simulink model "MarchMPC"  (R2024a)
settings: Solver=daessc  StartTime=0.0  StopTime=15  FixedStep=0.01  RelTol=1e-3
undefined symbols (not defined in the file): dw_des, leg_controller, LFstates, LRstates, model, p_cur, p_des, param, px, py, pz, Q, RFstates, RRstates, v_cur, v_des, vx, vy, vz, w, w_des, X, Y, Z
libraries: sm_lib x57, nesl_utility x47
(part 1 of 4)
settings Model: Creator=a123  LastModifiedBy=a123
settings RTWCC: GPUComputeCapability=3.5

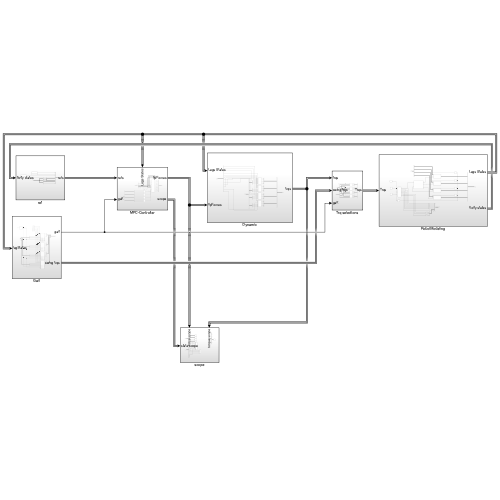
[thumbnail: Simulink's stored preview of the top-level diagram]
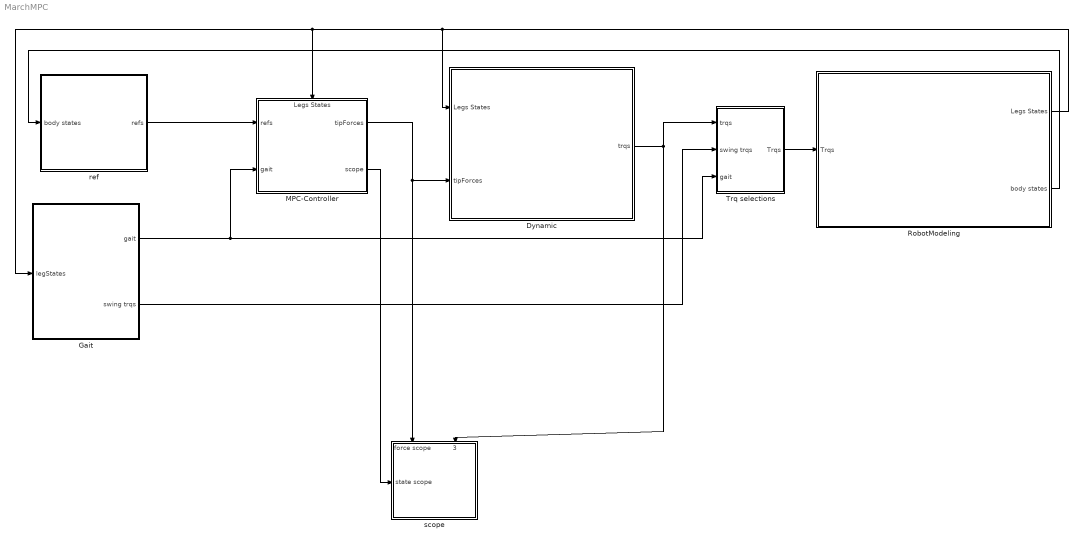
== system MarchMPC ==
  Dynamic : Subsystem
  Gait : Subsystem
  MPC-Controller : Subsystem
      settings: PortSchema="{\"entries\":[{\"content\":{\"sides\":[{\"content\":{\"connectorIds\":[\"In1\",\"In2\"]},\"type\":\"ConnectorPlacement.EquallySpacedRectSide\",\"uuid\":\"82207ac2-498d-428d-bb4d-b0457fff2070\"},{\"content\":{\"connectorIds\":[\"Out1\",\"Out2\"],\"side\":\"RIGHT\"},\"type\":\"ConnectorPlacement.EquallySpacedRectSide\",\"uuid\":\"62017463-8491-4b37-95c8-f619666068a7\"},{\"content\":{\"connectorIds\":[\"In3\"],\"side\":\"TOP\"},\"type\":\"ConnectorPlacement.EquallySpacedRectSide\",\"uuid\":\"cf9993cf-df0f-41a3-a963-d91c0f700b7a\"}]},\"type\":\"ConnectorPlacement.EquallySpacedConnector\",\"uuid\":\"3cbcd1c8-4438-4464-bb77-c195fb75fbb3\"}],\"packageUris\":[\"http://schema.mathworks.com/mf0/Connector/R2020b\"],\"version\":\"1.0\"}"
  RobotModeling : Subsystem
  Trq selections : Subsystem
  ref : Subsystem
  scope : Subsystem
      settings: PortSchema="{\"entries\":[{\"content\":{\"sides\":[{\"content\":{\"connectorIds\":[\"In1\"]},\"type\":\"ConnectorPlacement.EquallySpacedRectSide\",\"uuid\":\"c0265f70-bade-488b-ae2d-3c8d38e3d5ac\"},{\"content\":{\"side\":\"RIGHT\"},\"type\":\"ConnectorPlacement.EquallySpacedRectSide\",\"uuid\":\"4660b7bc-d16b-42a4-852b-cf8f48253a71\"},{\"content\":{\"connectorIds\":[\"In2\",\"In3\"],\"side\":\"TOP\"},\"type\":\"ConnectorPlacement.EquallySpacedRectSide\",\"uuid\":\"c4e122d6-8b41-4744-828b-3ddf3ee2b8ae\"}]},\"type\":\"ConnectorPlacement.EquallySpacedConnector\",\"uuid\":\"80d21178-9509-4fd6-959c-ba40dd2e55fa\"}],\"packageUris\":[\"http://schema.mathworks.com/mf0/Connector/R2020b\"],\"version\":\"1.0\"}"
  wires:
  RobotModeling/2(" body states") -> ref/1(body states)
  Dynamic/1(trqs) -> Trq selections/1(trqs), scope/3(torque scope)
  RobotModeling/1(Legs States) -> Dynamic/1(Legs States), MPC-Controller/3(Legs States), Gait/1(legStates)
  ref/1(refs) -> MPC-Controller/1(refs)
  Gait/1(gait) -> Trq selections/3(gait), MPC-Controller/2(gait)
  MPC-Controller/2(scope) -> scope/1(state scope)
  MPC-Controller/1(tipForces) -> Dynamic/2(tipForces), scope/2(force scope)
  Gait/2(swing trqs) -> Trq selections/2(swing trqs)
  Trq selections/1(Trqs) -> RobotModeling/1(Trqs)

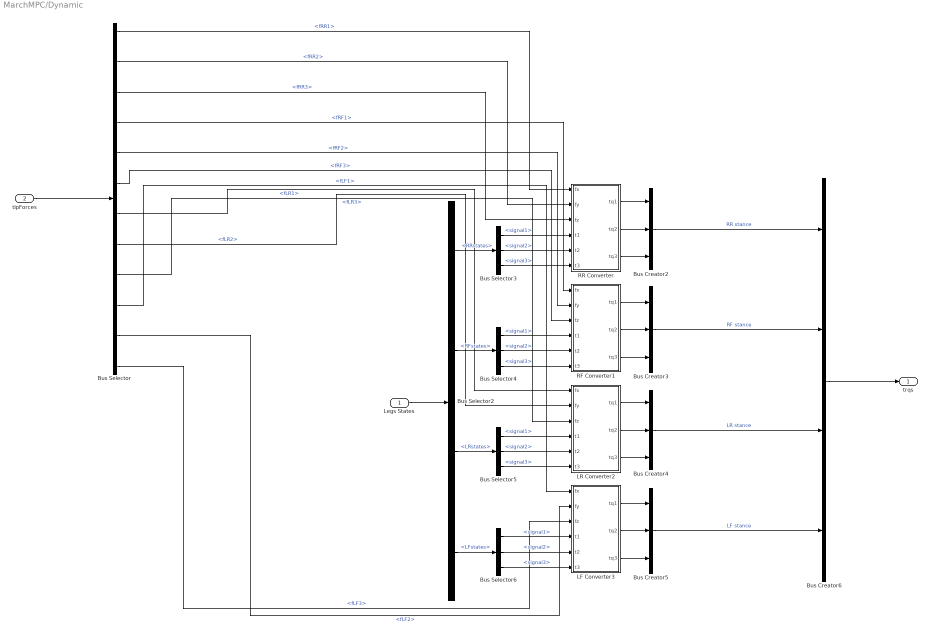
== system MarchMPC/Dynamic ==
  Legs States : Inport
  tipForces : Inport  Port=2
  Bus Creator{2..5} (4 alike) : BusCreator  Inputs=3
  Bus Creator6 : BusCreator  Inputs=4
  Bus Selector : BusSelector  OutputSignals=fRR1,fRR2,fRR3,fRF1,fRF2,fRF3,fLR1,fLR2,fLR3,fLF1,fLF2,fLF3
  Bus Selector2 : BusSelector  OutputSignals=RRstates,RFstates,LRstates,LFstates
  Bus Selector{3..6} (4 alike) : BusSelector  OutputSignals=signal1,signal2,signal3
  LF Converter3 : MATLAB Function  TreatAsAtomicUnit=on
  LR Converter2 : MATLAB Function  TreatAsAtomicUnit=on
  RF Converter1 : MATLAB Function  TreatAsAtomicUnit=on
  RR Converter : MATLAB Function  TreatAsAtomicUnit=on
  trqs : Outport
  wires:
  Bus Creator2/1 -> Bus Creator6/1  "RR stance"
  Bus Creator3/1 -> Bus Creator6/2  "RF stance"
  Bus Creator4/1 -> Bus Creator6/3  "LR stance"
  Bus Creator5/1 -> Bus Creator6/4  "LF stance"
  Bus Creator6/1 -> trqs/1
  Legs States/1 -> Bus Selector2/1
  Bus Selector2/1 -> Bus Selector3/1  "<RRstates>"
  Bus Selector3/1 -> RR Converter/4(t1)  "<signal1>"
  Bus Selector3/2 -> RR Converter/5(t2)  "<signal2>"
  Bus Selector3/3 -> RR Converter/6(t3)  "<signal3>"
  Bus Selector2/2 -> Bus Selector4/1  "<RFstates>"
  Bus Selector2/3 -> Bus Selector5/1  "<LRstates>"
  Bus Selector2/4 -> Bus Selector6/1  "<LFstates>"
  Bus Selector4/1 -> RF Converter1/4(t1)  "<signal1>"
  Bus Selector4/2 -> RF Converter1/5(t2)  "<signal2>"
  Bus Selector4/3 -> RF Converter1/6(t3)  "<signal3>"
  Bus Selector5/1 -> LR Converter2/4(t1)  "<signal1>"
  Bus Selector5/2 -> LR Converter2/5(t2)  "<signal2>"
  Bus Selector5/3 -> LR Converter2/6(t3)  "<signal3>"
  Bus Selector6/1 -> LF Converter3/4(t1)  "<signal1>"
  Bus Selector6/2 -> LF Converter3/5(t2)  "<signal2>"
  Bus Selector6/3 -> LF Converter3/6(t3)  "<signal3>"
  RR Converter/3(tq3) -> Bus Creator2/3
  RR Converter/2(tq2) -> Bus Creator2/2
  RR Converter/1(tq1) -> Bus Creator2/1
  RF Converter1/1(tq1) -> Bus Creator3/1
  RF Converter1/2(tq2) -> Bus Creator3/2
  RF Converter1/3(tq3) -> Bus Creator3/3
  LR Converter2/1(tq1) -> Bus Creator4/1
  LR Converter2/2(tq2) -> Bus Creator4/2
  LR Converter2/3(tq3) -> Bus Creator4/3
  LF Converter3/1(tq1) -> Bus Creator5/1
  LF Converter3/2(tq2) -> Bus Creator5/2
  LF Converter3/3(tq3) -> Bus Creator5/3
  tipForces/1 -> Bus Selector/1
  Bus Selector/1 -> RR Converter/1(fx)  "<fRR1>"
  Bus Selector/2 -> RR Converter/2(fy)  "<fRR2>"
  Bus Selector/3 -> RR Converter/3(fz)  "<fRR3>"
  Bus Selector/4 -> RF Converter1/1(fx)  "<fRF1>"
  Bus Selector/5 -> RF Converter1/2(fy)  "<fRF2>"
  Bus Selector/6 -> RF Converter1/3(fz)  "<fRF3>"
  Bus Selector/7 -> LR Converter2/1(fx)  "<fLR1>"
  Bus Selector/8 -> LR Converter2/2(fy)  "<fLR2>"
  Bus Selector/9 -> LR Converter2/3(fz)  "<fLR3>"
  Bus Selector/10 -> LF Converter3/1(fx)  "<fLF1>"
  Bus Selector/11 -> LF Converter3/2(fy)  "<fLF2>"
  Bus Selector/12 -> LF Converter3/3(fz)  "<fLF3>"

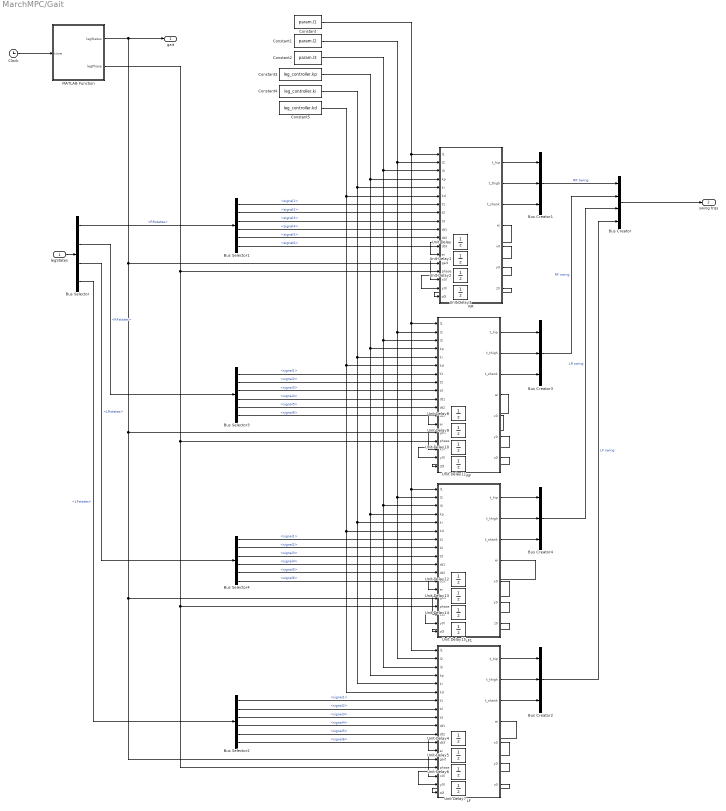
== system MarchMPC/Gait ==
  legStates : Inport
  Bus Creator : BusCreator  Inputs=RR Swing,RF swing,LR swing,LF swing
  Bus Creator{1..4} (4 alike) : BusCreator  Inputs=3
  Bus Selector : BusSelector  OutputSignals=RRstates,RFstates,LRstates,LFstates
  Bus Selector{1..4} (4 alike) : BusSelector  OutputSignals=signal1,signal2,signal3,signal4,signal5,signal6
  Clock : Clock
  Constant : Constant  Value=param.l1
  Constant1 : Constant  Value=param.l2
  Constant2 : Constant  Value=param.l3
  Constant3 : Constant  Value=leg_controller.kp
  Constant4 : Constant  Value=leg_controller.ki
  Constant5 : Constant  Value=leg_controller.kd
  LF : MATLAB Function  TreatAsAtomicUnit=on
  LF1 : MATLAB Function  TreatAsAtomicUnit=on
  MATLAB Function : MATLAB Function  TreatAsAtomicUnit=on
  RF : MATLAB Function  TreatAsAtomicUnit=on
  RR : MATLAB Function  TreatAsAtomicUnit=on
  Unit Delay{,4,8,12} (4 alike) : UnitDelay  InitialCondition=[0 0 0]  SampleTime=-1  HasFrameUpgradeWarning=on
  Unit Delay{1..3,5..7,9..11,13..15} (12 alike) : UnitDelay  SampleTime=-1  HasFrameUpgradeWarning=on
  gait : Outport
  swing trqs : Outport  Port=2
  wires:
  Clock/1 -> MATLAB Function/1(time)
  legStates/1 -> Bus Selector/1
  Bus Selector/1 -> Bus Selector1/1  "<RRstates>"
  RR/2(t_thigh) -> Bus Creator1/2
  RR/3(t_shank) -> Bus Creator1/3
  Bus Selector1/3 -> RR/9(t3)  "<signal3>"
  Bus Creator1/1 -> Bus Creator/1  "RR Swing"
  Bus Selector1/1 -> RR/7(t1)  "<signal1>"
  Bus Selector1/6 -> RR/12(dt3)  "<signal6>"
  Bus Selector1/5 -> RR/11(dt2)  "<signal5>"
  RR/1(t_hip) -> Bus Creator1/1
  Bus Selector1/2 -> RR/8(t2)  "<signal2>"
  Unit Delay/1 -> RR/13("ei ")
  Bus Selector1/4 -> RR/10(dt1)  "<signal4>"
  RR/4(ei) -> Unit Delay/1
  Bus Creator/1 -> swing trqs/1
  RR/5(x0) -> Unit Delay1/1
  Unit Delay1/1 -> RR/16(x0l)
  RR/6(y0) -> Unit Delay2/1
  Unit Delay2/1 -> RR/17(y0l)
  RR/7(z0) -> Unit Delay3/1
  Unit Delay3/1 -> RR/18(z0l)
  Unit Delay4/1 -> LF/13("ei ")
  LF/2(t_thigh) -> Bus Creator2/2
  LF/1(t_hip) -> Bus Creator2/1
  Unit Delay6/1 -> LF/17(y0l)
  LF/3(t_shank) -> Bus Creator2/3
  LF/4(ei) -> Unit Delay4/1
  Bus Creator2/1 -> Bus Creator/4  "LF swing"
  Bus Selector2/1 -> LF/7(t1)  "<signal1>"
  Bus Selector2/5 -> LF/11(dt2)  "<signal5>"
  Bus Selector2/2 -> LF/8(t2)  "<signal2>"
  Bus Selector2/3 -> LF/9(t3)  "<signal3>"
  LF/5(x0) -> Unit Delay5/1
  Bus Selector2/4 -> LF/10(dt1)  "<signal4>"
  Bus Selector2/6 -> LF/12(dt3)  "<signal6>"
  LF/6(y0) -> Unit Delay6/1
  Unit Delay7/1 -> LF/18(z0l)
  LF/7(z0) -> Unit Delay7/1
  Unit Delay5/1 -> LF/16(x0l)
  Bus Selector/4 -> Bus Selector2/1  "<LFstates>"
  Unit Delay8/1 -> RF/13("ei ")
  Bus Selector/2 -> Bus Selector3/1  "<RFstates>"
  Bus Selector3/1 -> RF/7(t1)  "<signal1>"
  RF/2(t_thigh) -> Bus Creator3/2
  RF/1(t_hip) -> Bus Creator3/1
  Unit Delay10/1 -> RF/17(y0l)
  MATLAB Function/1(legStatus) -> gait/1, LF/14(gait), LF1/14(gait), RF/14(gait), RR/14(gait)
  Bus Selector3/5 -> RF/11(dt2)  "<signal5>"
  MATLAB Function/2(legPhase) -> LF/15(phase), LF1/15(phase), RF/15(phase), RR/15(phase)
  Bus Selector3/2 -> RF/8(t2)  "<signal2>"
  Bus Selector3/3 -> RF/9(t3)  "<signal3>"
  RF/5(x0) -> Unit Delay9/1
  Bus Selector3/4 -> RF/10(dt1)  "<signal4>"
  RF/4(ei) -> Unit Delay8/1
  RF/3(t_shank) -> Bus Creator3/3
  Bus Selector3/6 -> RF/12(dt3)  "<signal6>"
  RF/6(y0) -> Unit Delay10/1
  Unit Delay11/1 -> RF/18(z0l)
  RF/7(z0) -> Unit Delay11/1
  Unit Delay9/1 -> RF/16(x0l)
  Bus Creator3/1 -> Bus Creator/2  "RF swing"
  Bus Selector/3 -> Bus Selector4/1  "<LRstates>"
  LF1/1(t_hip) -> Bus Creator4/1
  Unit Delay13/1 -> LF1/16(x0l)
  Unit Delay14/1 -> LF1/17(y0l)
  LF1/2(t_thigh) -> Bus Creator4/2
  Bus Selector4/1 -> LF1/7(t1)  "<signal1>"
  Bus Selector4/2 -> LF1/8(t2)  "<signal2>"
  Bus Selector4/3 -> LF1/9(t3)  "<signal3>"
  Unit Delay15/1 -> LF1/18(z0l)
  Bus Selector4/4 -> LF1/10(dt1)  "<signal4>"
  LF1/5(x0) -> Unit Delay13/1
  LF1/3(t_shank) -> Bus Creator4/3
  LF1/4(ei) -> Unit Delay12/1
  LF1/7(z0) -> Unit Delay15/1
  LF1/6(y0) -> Unit Delay14/1
  Bus Selector4/6 -> LF1/12(dt3)  "<signal6>"
  Bus Selector4/5 -> LF1/11(dt2)  "<signal5>"
  Unit Delay12/1 -> LF1/13("ei ")
  Bus Creator4/1 -> Bus Creator/3  "LR swing"
  Constant/1 -> RR/1(l1), LF/1(l1), LF1/1(l1), RF/1(l1)
  Constant1/1 -> RR/2(l2), LF/2(l2), LF1/2(l2), RF/2(l2)
  Constant2/1 -> RR/3(l3), LF/3(l3), LF1/3(l3), RF/3(l3)
  Constant3/1 -> LF/4(kp), LF1/4(kp), RF/4(kp), RR/4(kp)
  Constant4/1 -> LF/5(ki), LF1/5(ki), RF/5(ki), RR/5(ki)
  Constant5/1 -> LF/6(kd), LF1/6(kd), RF/6(kd), RR/6(kd)

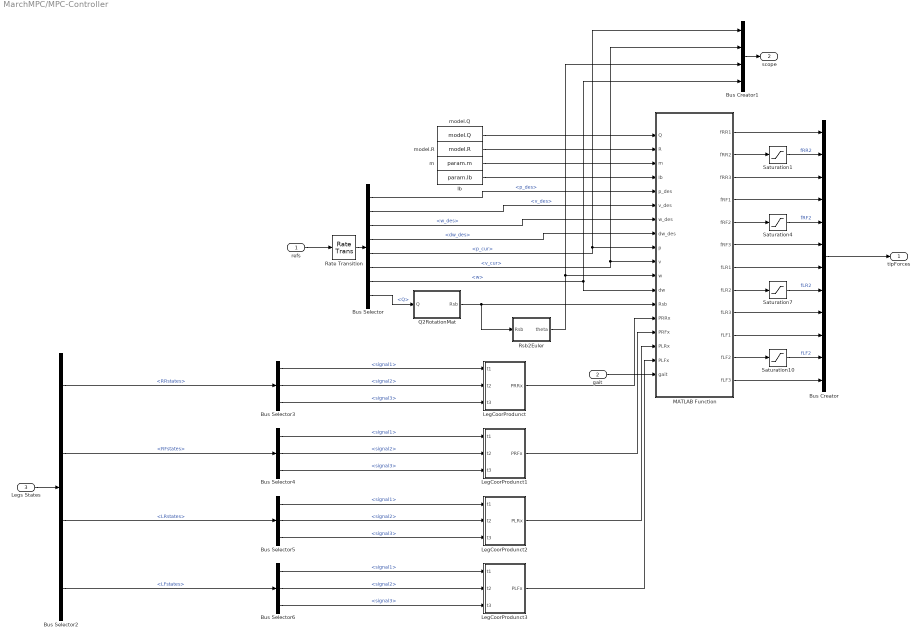
== system MarchMPC/MPC-Controller ==
  refs : Inport
  gait : Inport  Port=2
  Legs States : Inport  Port=3
  Bus Creator : BusCreator  Inputs=12
  Bus Creator1 : BusCreator  Inputs=4
  Bus Selector : BusSelector  OutputSignals=p_des,v_des,w_des,dw_des,p_cur,v_cur,w,Q
  Bus Selector2 : BusSelector  OutputSignals=RRstates,RFstates,LRstates,LFstates
  Bus Selector{3..6} (4 alike) : BusSelector  OutputSignals=signal1,signal2,signal3
  Ib : Constant  Value=param.Ib  VectorParams1D=off
  LegCoorProdunct : MATLAB Function  TreatAsAtomicUnit=on
  LegCoorProdunct1 : MATLAB Function  TreatAsAtomicUnit=on
  LegCoorProdunct2 : MATLAB Function  TreatAsAtomicUnit=on
  LegCoorProdunct3 : MATLAB Function  TreatAsAtomicUnit=on
  MATLAB Function : MATLAB Function  TreatAsAtomicUnit=on
  Q2RotationMat : MATLAB Function  TreatAsAtomicUnit=on
  Rate Transition : RateTransition  OutPortSampleTime=0.01
  Rsb2Euler : MATLAB Function  TreatAsAtomicUnit=on
  Saturation{1,4,7,10} (4 alike) : Saturate  UpperLimit=200  LowerLimit=0
  m : Constant  Value=param.m
  model.Q : Constant  Value=model.Q  VectorParams1D=off
  model.R : Constant  Value=model.R  VectorParams1D=off
  tipForces : Outport
  scope : Outport  Port=2
  wires:
  refs/1 -> Rate Transition/1
  Bus Selector/1 -> MATLAB Function/5(p_des)  "<p_des>"
  Bus Selector/2 -> MATLAB Function/6(v_des)  "<v_des>"
  Bus Selector/3 -> MATLAB Function/7(w_des)  "<w_des>"
  Bus Selector/4 -> MATLAB Function/8(dw_des)  "<dw_des>"
  Bus Selector/5 -> Bus Creator1/1, MATLAB Function/9(p)  "<p_cur>"
  Bus Selector/6 -> Bus Creator1/2, MATLAB Function/10(v)  "<v_cur>"
  Bus Selector/7 -> Bus Creator1/4, MATLAB Function/12(dw)  "<w>"
  Bus Selector/8 -> Q2RotationMat/1(Q)  "<Q>"
  Bus Selector5/2 -> LegCoorProdunct2/2(t2)  "<signal2>"
  Bus Selector5/3 -> LegCoorProdunct2/3(t3)  "<signal3>"
  Bus Selector6/3 -> LegCoorProdunct3/3(t3)  "<signal3>"
  Bus Selector2/3 -> Bus Selector5/1  "<LRstates>"
  Bus Selector6/1 -> LegCoorProdunct3/1(t1)  "<signal1>"
  Bus Selector4/2 -> LegCoorProdunct1/2(t2)  "<signal2>"
  Bus Selector6/2 -> LegCoorProdunct3/2(t2)  "<signal2>"
  Bus Selector3/2 -> LegCoorProdunct/2(t2)  "<signal2>"
  Bus Selector5/1 -> LegCoorProdunct2/1(t1)  "<signal1>"
  Bus Selector2/2 -> Bus Selector4/1  "<RFstates>"
  Bus Selector2/1 -> Bus Selector3/1  "<RRstates>"
  Legs States/1 -> Bus Selector2/1
  Bus Selector3/3 -> LegCoorProdunct/3(t3)  "<signal3>"
  Bus Selector4/1 -> LegCoorProdunct1/1(t1)  "<signal1>"
  Bus Selector3/1 -> LegCoorProdunct/1(t1)  "<signal1>"
  Bus Selector4/3 -> LegCoorProdunct1/3(t3)  "<signal3>"
  Bus Selector2/4 -> Bus Selector6/1  "<LFstates>"
  Bus Creator/1 -> tipForces/1
  Q2RotationMat/1(Rsb) -> Rsb2Euler/1(Rsb), MATLAB Function/13(Rsb)
  m/1 -> MATLAB Function/3(m)
  Ib/1 -> MATLAB Function/4(Ib)
  LegCoorProdunct/1(PRRx) -> MATLAB Function/14(PRRx)
  LegCoorProdunct1/1(PRFx) -> MATLAB Function/15(PRFx)
  LegCoorProdunct2/1(PLRx) -> MATLAB Function/16(PLRx)
  LegCoorProdunct3/1(PLFx) -> MATLAB Function/17(PLFx)
  Rate Transition/1 -> Bus Selector/1
  Rsb2Euler/1(theta) -> Bus Creator1/3, MATLAB Function/11(w)
  Bus Creator1/1 -> scope/1
  gait/1 -> MATLAB Function/18(gait)
  MATLAB Function/1(fRR1) -> Bus Creator/1
  MATLAB Function/2(fRR2) -> Saturation1/1
  MATLAB Function/5(fRF2) -> Saturation4/1
  MATLAB Function/8(fLR2) -> Saturation7/1
  MATLAB Function/11(fLF2) -> Saturation10/1
  Saturation1/1 -> Bus Creator/2  "fRR2"
  MATLAB Function/3(fRR3) -> Bus Creator/3
  MATLAB Function/4(fRF1) -> Bus Creator/4
  Saturation4/1 -> Bus Creator/5  "fRF2"
  MATLAB Function/6(fRF3) -> Bus Creator/6
  MATLAB Function/7(fLR1) -> Bus Creator/7
  Saturation7/1 -> Bus Creator/8  "fLR2"
  MATLAB Function/9(fLR3) -> Bus Creator/9
  MATLAB Function/10(fLF1) -> Bus Creator/10
  Saturation10/1 -> Bus Creator/11  "fLF2"
  MATLAB Function/12(fLF3) -> Bus Creator/12
  model.Q/1 -> MATLAB Function/1(Q)
  model.R/1 -> MATLAB Function/2(R)

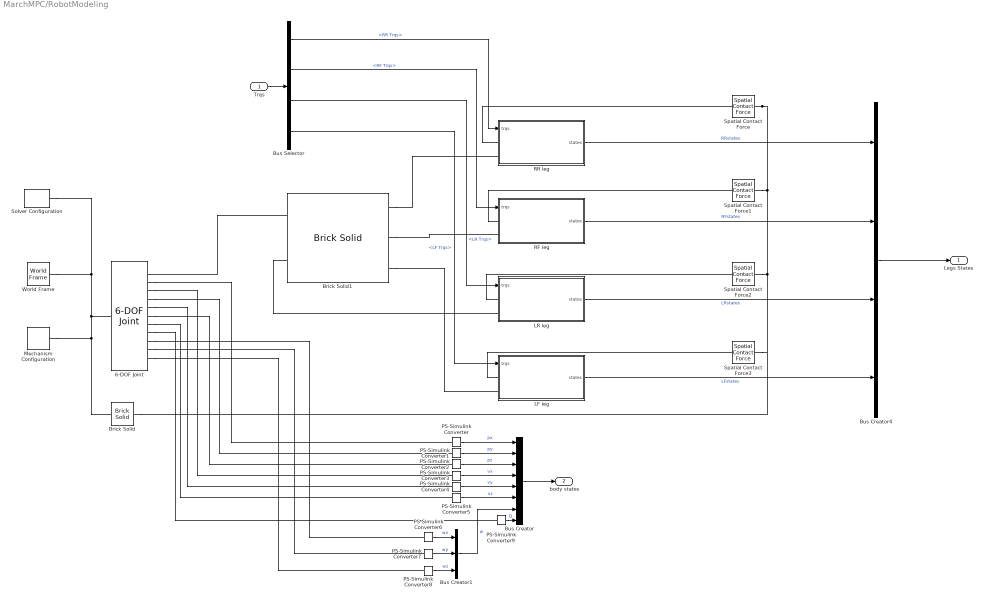
== system MarchMPC/RobotModeling ==
  Trqs : Inport
  6-DOF Joint : sm_lib/Joints/6-DOF Joint  JointMode=Normal  CompositeWrenchDir=FollowerOnBase  CompositeWrenchFrame=BaseFrame  SenseConstraintForce=off  SenseConstraintTorque=off  SenseTotalForce=off  SenseTotalTorque=off  PxPositionTargetSpecify=off  PxPositionTargetPriority=High  PxPositionTargetValue=0  PxPositionTargetValueUnits=m  PxVelocityTargetSpecify=off  PxVelocityTargetPriority=High  PxVelocityTargetValue=0  PxVelocityTargetValueUnits=m/s  PxEquilibriumPosition=0  PxEquilibriumPositionUnits=m  PxSpringStiffness=0  PxSpringStiffnessUnits=N/m  PxDampingCoefficient=0  PxDampingCoefficientUnits=N/(m/s)  PxLowerLimitSpecify=off  PxLowerLimitBound=-1  PxLowerLimitBoundUnits=m  PxLowerLimitStiffness=1e6  PxLowerLimitStiffnessUnits=N/m  PxLowerLimitDamping=1e3  PxLowerLimitDampingUnits=N/(m/s)  PxLowerLimitTransitionRegionWidth=1e-4  PxLowerLimitTransitionRegionWidthUnits=m  PxUpperLimitSpecify=off  PxUpperLimitBound=1  PxUpperLimitBoundUnits=m  PxUpperLimitStiffness=1e6  PxUpperLimitStiffnessUnits=N/m  PxUpperLimitDamping=1e3  PxUpperLimitDampingUnits=N/(m/s)  PxUpperLimitTransitionRegionWidth=1e-4  PxUpperLimitTransitionRegionWidthUnits=m  PxTorqueActuationMode=NoTorque  PxMotionActuationMode=ComputedMotion  PxSensePosition=on  PxSenseVelocity=on  PxSenseAcceleration=off  PxSenseTorqueForce=off  PxSenseLowerLimitTorqueForce=off  PxSenseUpperLimitTorqueForce=off  PyPositionTargetSpecify=on  PyPositionTargetPriority=High  PyPositionTargetValue=1.22  PyPositionTargetValueUnits=m  PyVelocityTargetSpecify=off  PyVelocityTargetPriority=High  PyVelocityTargetValue=0  PyVelocityTargetValueUnits=m/s  PyEquilibriumPosition=0  PyEquilibriumPositionUnits=m  PySpringStiffness=0  PySpringStiffnessUnits=N/m  PyDampingCoefficient=0  PyDampingCoefficientUnits=N/(m/s)  PyLowerLimitSpecify=off  PyLowerLimitBound=-1  PyLowerLimitBoundUnits=m  PyLowerLimitStiffness=1e6  PyLowerLimitStiffnessUnits=N/m  PyLowerLimitDamping=1e3  PyLowerLimitDampingUnits=N/(m/s)  PyLowerLimitTransitionRegionWidth=1e-4  PyLowerLimitTransitionRegionWidthUnits=m  PyUpperLimitSpecify=off  PyUpperLimitBound=1  PyUpperLimitBoundUnits=m  PyUpperLimitStiffness=1e6  PyUpperLimitStiffnessUnits=N/m  PyUpperLimitDamping=1e3  PyUpperLimitDampingUnits=N/(m/s)  PyUpperLimitTransitionRegionWidth=1e-4  PyUpperLimitTransitionRegionWidthUnits=m  PyTorqueActuationMode=NoTorque  PyMotionActuationMode=ComputedMotion  PySensePosition=on  PySenseVelocity=on  PySenseAcceleration=off  PySenseTorqueForce=off  PySenseLowerLimitTorqueForce=off  PySenseUpperLimitTorqueForce=off  PzPositionTargetSpecify=off  PzPositionTargetPriority=High  PzPositionTargetValue=0  PzPositionTargetValueUnits=m  PzVelocityTargetSpecify=off  PzVelocityTargetPriority=High  PzVelocityTargetValue=0  PzVelocityTargetValueUnits=m/s  PzEquilibriumPosition=0  PzEquilibriumPositionUnits=m  PzSpringStiffness=0  PzSpringStiffnessUnits=N/m  PzDampingCoefficient=0  PzDampingCoefficientUnits=N/(m/s)  PzLowerLimitSpecify=off  PzLowerLimitBound=-1  PzLowerLimitBoundUnits=m  PzLowerLimitStiffness=1e6  PzLowerLimitStiffnessUnits=N/m  PzLowerLimitDamping=1e3  PzLowerLimitDampingUnits=N/(m/s)  PzLowerLimitTransitionRegionWidth=1e-4  PzLowerLimitTransitionRegionWidthUnits=m  PzUpperLimitSpecify=off  PzUpperLimitBound=1  PzUpperLimitBoundUnits=m  PzUpperLimitStiffness=1e6  PzUpperLimitStiffnessUnits=N/m  PzUpperLimitDamping=1e3  PzUpperLimitDampingUnits=N/(m/s)  PzUpperLimitTransitionRegionWidth=1e-4  PzUpperLimitTransitionRegionWidthUnits=m  PzTorqueActuationMode=NoTorque  PzMotionActuationMode=ComputedMotion  PzSensePosition=on  PzSenseVelocity=on  PzSenseAcceleration=off  PzSenseTorqueForce=off  PzSenseLowerLimitTorqueForce=off  PzSenseUpperLimitTorqueForce=off  SphPositionTargetSpecify=off  SphPositionTargetPriority=High  SphPositionTargetRotationMethod=Quaternion  SphPositionTargetFollAlignAxisA=+X  SphPositionTargetBaseAlignAxisA=+Y  SphPositionTargetFollAlignAxisB=+Y  SphPositionTargetBaseAlignAxisB=+Z  SphPositionTargetRotationStandardAxis=+Z  SphPositionTargetRotationAngle=0.0  SphPositionTargetRotationAngleUnits=deg  SphPositionTargetRotationArbitraryAxis=[0 0 1]  SphPositionTargetRotationSequenceAxes=FollowerAxes  SphPositionTargetRotationSequence=XYX  SphPositionTargetRotationSequenceAngles=[0 0 0]  SphPositionTargetRotationSequenceAnglesUnits=deg  SphPositionTargetRotationMatrix=[1 0 0; 0 1 0; 0 0 1]  SphPositionTargetQuaternion=[0.9 0 0 0]  SphVelocityTargetSpecify=off  SphVelocityTargetPriority=High  SphVelocityTargetValue=[0 0 0]  SphVelocityTargetValueUnits=deg/s  SphVelocityTargetInFollowerFrame=on  SphEqPosRotationMethod=None  SphEqPosFollAlignAxisA=+X  SphEqPosBaseAlignAxisA=+Y  SphEqPosFollAlignAxisB=+Y  SphEqPosBaseAlignAxisB=+Z  SphEqPosRotationStandardAxis=+Z  SphEqPosRotationAngle=0.0  SphEqPosRotationAngleUnits=deg  SphEqPosRotationArbitraryAxis=[0 0 1]  SphEqPosRotationSequenceAxes=FollowerAxes  SphEqPosRotationSequence=XYX  SphEqPosRotationSequenceAngles=[0 0 0]  SphEqPosRotationSequenceAnglesUnits=deg  SphEqPosRotationMatrix=[1 0 0; 0 1 0; 0 0 1]  SphEqPosQuaternion=[1 0 0 0]  SphSpringStiffness=0  SphSpringStiffnessUnits=N*m/deg  SphDampingCoefficient=0  SphDampingCoefficientUnits=N*m/(deg/s)  SphLowerLimitSpecify=off  SphLowerLimitBound=15  SphLowerLimitBoundUnits=deg  SphLowerLimitStiffness=1e4  SphLowerLimitStiffnessUnits=N*m/deg  SphLowerLimitDamping=10  SphLowerLimitDampingUnits=N*m/(deg/s)  SphLowerLimitTransitionRegionWidth=0.1  SphLowerLimitTransitionRegionWidthUnits=deg  SphUpperLimitSpecify=off  SphUpperLimitBound=45  SphUpperLimitBoundUnits=deg  SphUpperLimitStiffness=1e4  SphUpperLimitStiffnessUnits=N*m/deg  SphUpperLimitDamping=10  SphUpperLimitDampingUnits=N*m/(deg/s)  SphUpperLimitTransitionRegionWidth=0.1  SphUpperLimitTransitionRegionWidthUnits=deg  SphTorqueActuationMode=NoTorque  SphActuateTorqueX=off  SphActuateTorqueY=off  SphActuateTorqueZ=off  SphActuateTorque=off  SphActuationFrame=BaseFrame  SphSensePosition=on  SphSenseVelocityX=on  SphSenseVelocityY=on  SphSenseVelocityZ=on  SphSenseVelocity=off  SphSenseAccelerationX=off  SphSenseAccelerationY=off  SphSenseAccelerationZ=off  SphSenseAcceleration=off  SphSenseLowerLimitTorqueMag=off  SphSenseUpperLimitTorqueMag=off  SphSensingFrame=BaseFrame
  Brick Solid : sm_lib/Body Elements/Brick Solid  BrickDimensions=[20 0.01 20]  BrickDimensionsUnits=m  ExportEntireGeometry=on  InertiaType=CalculateFromGeometry  BasedOnType=Density  Density=1000  DensityUnits=kg/m^3  Mass=1  MassUnits=kg  CenterOfMass=[0 0 0]  CenterOfMassUnits=m  MomentsOfInertia=[1 1 1]  MomentsOfInertiaUnits=kg*m^2  ProductsOfInertia=[0 0 0]  ProductsOfInertiaUnits=kg*m^2  GraphicType=FromGeometry  MarkerShape=Sphere  MarkerSize=10  GraphicVisPropType=SimpleVisualProperties  GraphicDiffuseColor=[0.5 0.5 0.5]  GraphicOpacity=1.0  GraphicSpecularColor=[0.5 0.5 0.5 1.0]  GraphicAmbientColor=[0.15 0.15 0.15 1.0]  GraphicEmissiveColor=[0.0 0.0 0.0 1.0]  GraphicShininess=75  DoExposeReferenceFrame=on  SerializedFrames=<Frames/>
  Brick Solid1 : sm_lib/Body Elements/Brick Solid  BrickDimensions=[2.5 0.3 0.8]  BrickDimensionsUnits=m  ExportEntireGeometry=off  InertiaType=Custom  BasedOnType=Mass  Density=1000  DensityUnits=kg/m^3  Mass=20  MassUnits=kg  CenterOfMass=[0 0 0]  CenterOfMassUnits=m  MomentsOfInertia=[5 5 5]  MomentsOfInertiaUnits=kg*m^2  ProductsOfInertia=[0 0 0]  ProductsOfInertiaUnits=kg*m^2  GraphicType=FromGeometry  MarkerShape=Sphere  MarkerSize=10  GraphicVisPropType=SimpleVisualProperties  GraphicDiffuseColor=[1.0 0.6 0.2]  GraphicOpacity=1.0  GraphicSpecularColor=[0.5 0.5 0.5 1.0]  GraphicAmbientColor=[0.15 0.15 0.15 1.0]  GraphicEmissiveColor=[0.0 0.0 0.0 1.0]  GraphicShininess=75  DoExposeReferenceFrame=on  SerializedFrames=<Frames><Frame><Id>Frame1</Id><Value><Name>RR</Name><Origin><Source>ReferenceFrame</Source><FeatureName></FeatureName></Origin><PrimaryAxis><DefinedDirection>+Z</DefinedDirection><Source>ReferenceFrame</Source><SourceDirection>-X</SourceDirection><FeatureName></FeatureName></PrimaryAxis><SecondaryAxis><DefinedDirection>+X</DefinedDirection><Source>ReferenceFrame</Source><SourceDirection>+Z</SourceDirection><FeatureName></FeatureName></SecondaryAxis></Value></Frame><Frame><Id>Frame2</Id><Value><Name>RF</Name><Origin><Source>ReferenceFrame</Source><FeatureName></FeatureName></Origin><PrimaryAxis><DefinedDirection>+Z</DefinedDirection><Source>ReferenceFrame</Source><SourceDirection>-X</SourceDirection><FeatureName></FeatureName></PrimaryAxis><SecondaryAxis><DefinedDirection>+X</DefinedDirection><Source>ReferenceFrame</Source><SourceDirection>+Z</SourceDirection><FeatureName></FeatureName></SecondaryAxis></Value></Frame><Frame><Id>Frame3</Id><Value><Name>LR</Name><Origin><Source>ReferenceFrame</Source><FeatureName></FeatureName></Origin><PrimaryAxis><DefinedDirection>+Z</DefinedDirection><Source>ReferenceFrame</Source><SourceDirection>-X</SourceDirection><FeatureName></FeatureName></PrimaryAxis><SecondaryAxis><DefinedDirection>+X</DefinedDirection><Source>ReferenceFrame</Source><SourceDirection>+Z</SourceDirection><FeatureName></FeatureName></SecondaryAxis></Value></Frame><Frame><Id>Frame4</Id><Value><Name>LF</Name><Origin><Source>ReferenceFrame</Source><FeatureName></FeatureName></Origin><PrimaryAxis><DefinedDirection>+Z</DefinedDirection><Source>ReferenceFrame</Source><SourceDirection>-X</SourceDirection><FeatureName></FeatureName></PrimaryAxis><SecondaryAxis><DefinedDirection>+X</DefinedDirection><Source>ReferenceFrame</Source><SourceDirection>+Z</SourceDirection><FeatureName></FeatureName></SecondaryAxis></Value></Frame></Frames>
  Bus Creator : BusCreator  Inputs=px,py,pz,vx,vy,vz,w,Q
  Bus Creator1 : BusCreator  Inputs=3
  Bus Creator4 : BusCreator  Inputs=RRstates,RFstates,LRstates,LFstates
  Bus Selector : BusSelector  OutputSignals=RR Trqs,RF Trqs,LR Trqs,LF Trqs
  LF leg : Subsystem
  LR leg : Subsystem
  Mechanism Configuration : sm_lib/Utilities/Mechanism Configuration  UniformGravity=Constant  GravityVector=[0 -9.80665 0]  GravityVectorUnits=m/s^2  LinearizationDelta=0.001  JointModeTransitionNonlinearIterations=2
  PS-Simulink Converter{,1..9} (10 alike) : nesl_utility/PS-Simulink Converter  PhysicalDomain=network_engine_domain  SubClassName=ps_output  LeftPortType=input  RightPortType=output  PseudoPeriodic=off  Frequencies=[]  VectorFormat=inherit  Unit=inherit  AffineConversion=off
  RF leg : Subsystem
  RR leg : Subsystem
  Solver Configuration : nesl_utility/Solver Configuration  PhysicalDomain=network_engine_domain  SubClassName=solver  LeftPortType=input  RightPortType=generic  Tones=[]  Harmonics=[]  SimulateNoise=off  Profile=off  UseLocalSampling=off  EnableSwitchedLinearOptims=on  FrequencyDomain=off  UseCCode=off  RelTol=0.001  AbsTol=0.001  MinStep=1e-09  ToWorkspace=off  RevertToSquareIcSolve=off  NumHomotopyIterations=100  PhasorMode=off  PhasorModeNumHarmonics=1  ConsistencySolver=NEWTON_XTOL_AFTER_FTOL  IndexReductionMethod=DerivativeReplacement  DoDC=off  ResidualTolerance=1e-09  ConsistencyTolSource=GLOBAL  ConsistencyAbsTol=0.001  ConsistencyRelTol=0.001  ConsistencyTolFactor=0.001  UseLocalSolver=off  LocalSolverChoice=NE_BACKWARD_EULER_ADVANCER  ResolveIndetEquations=on  FunctionEvalNumThread=1  LocalSolverSampleTime=0.001  DoFixedCost=off  MaxNonlinIter=3  MaxModeIter=2  ComputeImpulses=off  ImpulseIterations=2  LinearAlgebra=auto  LinearAlgebraNumThread=0  EquationFormulation=NE_TIME_EF  DelaysMemoryBudget=1024  AutomaticFiltering=on  FilteringTimeConstant=0.001  PartitionStorageMethod=AS_NEEDED  PartitionMemoryBudget=1024  PartitionMethod=ROBUST  MultibodyUseLocalSolver=off  MultibodyLocalSolverChoice=ODE1  MultibodyLocalSolverSampleTime=0.001
  Spatial Contact Force{,1..3} (4 alike) : sm_lib/Forces and Torques/Spatial Contact Force  NormalForceType=SmoothSpringDamper  NormalStiffness=1e6  NormalStiffnessUnits=N/m  NormalDamping=1e3  NormalDampingUnits=N/(m/s)  NormalTransitionRegionWidth=1e-4  NormalTransitionRegionWidthUnits=m  FrictionType=SmoothStickSlip  CoefficientOfStaticFriction=2  CoefficientOfDynamicFriction=2  FrictionalCriticalVelocity=1e-3  FrictionalCriticalVelocityUnits=m/s  SenseContactSignal=off  SensePenetrationDepth=off  SenseSeparationDistance=off  SenseNormalForceMagnitude=off  SenseFrictionalForceMagnitude=off  SenseNormalVelocity=off  SenseTangentialVelocity=off  SenseContactBaseRotation=off  SenseContactBaseTranslation=off  SenseContactFollowerRotation=off  SenseContactFollowerTranslation=off  ZeroCrossDetectContactStartAndEnd=off
  World Frame : sm_lib/Frames and Transforms/World Frame
  Legs States : Outport
  " body states" : Outport  Port=2
  wires:
  Bus Creator4/1 -> Legs States/1
  RR leg/1(states) -> Bus Creator4/1  "RRstates"
  RF leg/1(states) -> Bus Creator4/2  "RFstates"
  LR leg/1(states) -> Bus Creator4/3  "LRstates"
  LF leg/1(states) -> Bus Creator4/4  "LFstates"
  PS-Simulink Converter/1 -> Bus Creator/1  "px"
  PS-Simulink Converter1/1 -> Bus Creator/2  "py"
  PS-Simulink Converter2/1 -> Bus Creator/3  "pz"
  PS-Simulink Converter3/1 -> Bus Creator/4  "vx"
  PS-Simulink Converter4/1 -> Bus Creator/5  "vy"
  PS-Simulink Converter5/1 -> Bus Creator/6  "vz"
  Bus Creator/1 -> " body states"/1
  PS-Simulink Converter8/1 -> Bus Creator1/3  "wz"
  PS-Simulink Converter7/1 -> Bus Creator1/2  "wy"
  PS-Simulink Converter6/1 -> Bus Creator1/1  "wx"
  Bus Creator1/1 -> Bus Creator/7  "w"
  PS-Simulink Converter9/1 -> Bus Creator/8  "Q"
  Trqs/1 -> Bus Selector/1
  Bus Selector/4 -> LF leg/1(trqs)  "<LF Trqs>"
  Bus Selector/3 -> LR leg/1(trqs)  "<LR Trqs>"
  Bus Selector/2 -> RF leg/1(trqs)  "<RF Trqs>"
  Bus Selector/1 -> RR leg/1(trqs)  "<RR Trqs>"
  connections:
  Solver Configuration/RConn1 -- Mechanism Configuration/RConn1 -- Brick Solid/RConn1 -- 6-DOF Joint/LConn1 -- World Frame/RConn1
  Brick Solid1/RConn1 -- 6-DOF Joint/RConn1
  Spatial Contact Force/LConn1 -- RR leg/LConn1
  Spatial Contact Force/RConn1 -- Spatial Contact Force3/RConn1 -- Brick Solid/LConn1 -- Spatial Contact Force2/RConn1 -- Spatial Contact Force1/RConn1
  Brick Solid1/LConn1 -- RR leg/LConn2
  Brick Solid1/LConn2 -- RF leg/LConn2
  Brick Solid1/LConn3 -- LF leg/LConn2
  Brick Solid1/RConn2 -- LR leg/LConn2
  Spatial Contact Force1/LConn1 -- RF leg/LConn1
  Spatial Contact Force2/LConn1 -- LR leg/LConn1
  Spatial Contact Force3/LConn1 -- LF leg/LConn1
  6-DOF Joint/RConn2 -- PS-Simulink Converter/LConn1
  6-DOF Joint/RConn4 -- PS-Simulink Converter1/LConn1
  6-DOF Joint/RConn6 -- PS-Simulink Converter2/LConn1
  6-DOF Joint/RConn3 -- PS-Simulink Converter3/LConn1
  6-DOF Joint/RConn5 -- PS-Simulink Converter4/LConn1
  6-DOF Joint/RConn7 -- PS-Simulink Converter5/LConn1
  6-DOF Joint/RConn9 -- PS-Simulink Converter6/LConn1
  6-DOF Joint/RConn10 -- PS-Simulink Converter7/LConn1
  6-DOF Joint/RConn11 -- PS-Simulink Converter8/LConn1
  6-DOF Joint/RConn8 -- PS-Simulink Converter9/LConn1

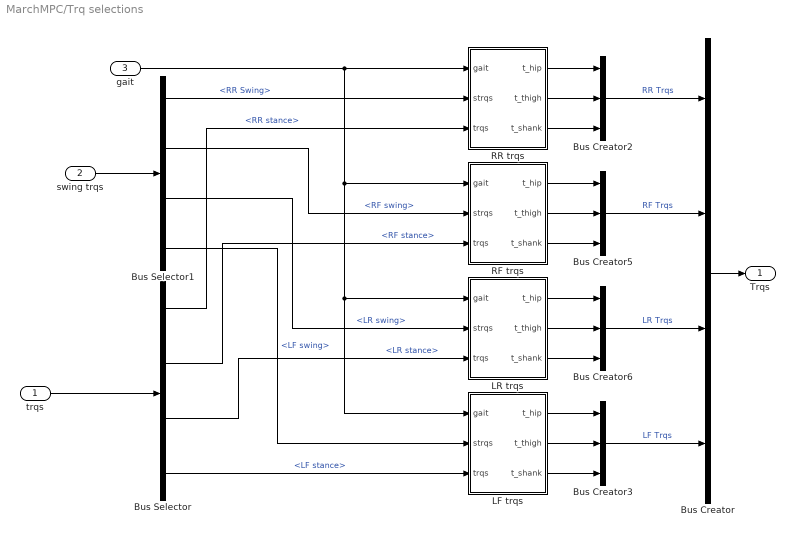
== system MarchMPC/Trq selections ==
  trqs : Inport
  swing trqs : Inport  Port=2
  gait : Inport  Port=3
  Bus Creator : BusCreator  Inputs=RR Trqs,RF Trqs,LR Trqs,LF Trqs
  Bus Creator{2..3,5..6} (4 alike) : BusCreator  Inputs=3
  Bus Selector : BusSelector  OutputSignals=RR stance,RF stance,LR stance,LF stance
  Bus Selector1 : BusSelector  OutputSignals=RR Swing,RF swing,LR swing,LF swing
  LF trqs : MATLAB Function  TreatAsAtomicUnit=on
  LR trqs : MATLAB Function  TreatAsAtomicUnit=on
  RF trqs : MATLAB Function  TreatAsAtomicUnit=on
  RR trqs : MATLAB Function  TreatAsAtomicUnit=on
  Trqs : Outport
  wires:
  LR trqs/3(t_shank) -> Bus Creator6/3
  Bus Selector/3 -> LR trqs/3(trqs)  "<LR stance>"
  Bus Selector1/2 -> RF trqs/2(strqs)  "<RF swing>"
  RR trqs/2(t_thigh) -> Bus Creator2/2
  LR trqs/1(t_hip) -> Bus Creator6/1
  RR trqs/3(t_shank) -> Bus Creator2/3
  LF trqs/3(t_shank) -> Bus Creator3/3
  RF trqs/1(t_hip) -> Bus Creator5/1
  RF trqs/2(t_thigh) -> Bus Creator5/2
  LR trqs/2(t_thigh) -> Bus Creator6/2
  LF trqs/2(t_thigh) -> Bus Creator3/2
  RF trqs/3(t_shank) -> Bus Creator5/3
  LF trqs/1(t_hip) -> Bus Creator3/1
  Bus Selector/2 -> RF trqs/3(trqs)  "<RF stance>"
  Bus Selector1/3 -> LR trqs/2(strqs)  "<LR swing>"
  gait/1 -> RF trqs/1(gait), LR trqs/1(gait), LF trqs/1(gait), RR trqs/1(gait)
  swing trqs/1 -> Bus Selector1/1
  Bus Selector/1 -> RR trqs/3(trqs)  "<RR stance>"
  RR trqs/1(t_hip) -> Bus Creator2/1
  Bus Selector1/1 -> RR trqs/2(strqs)  "<RR Swing>"
  Bus Selector/4 -> LF trqs/3(trqs)  "<LF stance>"
  trqs/1 -> Bus Selector/1
  Bus Selector1/4 -> LF trqs/2(strqs)  "<LF swing>"
  Bus Creator/1 -> Trqs/1
  Bus Creator2/1 -> Bus Creator/1  "RR Trqs"
  Bus Creator5/1 -> Bus Creator/2  "RF Trqs"
  Bus Creator6/1 -> Bus Creator/3  "LR Trqs"
  Bus Creator3/1 -> Bus Creator/4  "LF Trqs"

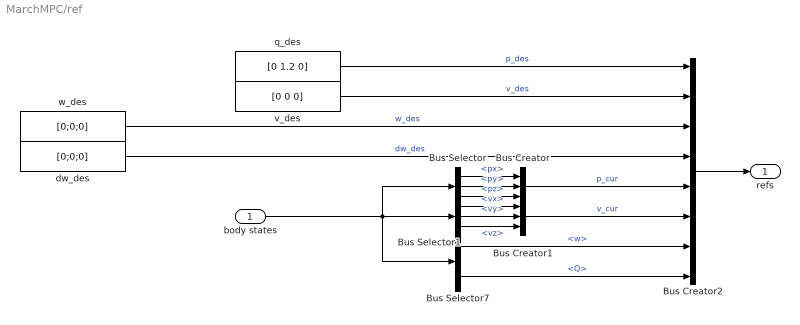
== system MarchMPC/ref ==
  body states : Inport
  Bus Creator : BusCreator  Inputs=3
  Bus Creator1 : BusCreator  Inputs=3
  Bus Creator2 : BusCreator  Inputs=p_des,v_des,w_des,dw_des,p_cur,v_cur,w,Q
  Bus Selector : BusSelector  OutputSignals=px,py,pz
  Bus Selector1 : BusSelector  OutputSignals=vx,vy,vz
  Bus Selector7 : BusSelector  OutputSignals=w,Q
  dw_des : Constant  Value=[0;0;0]  VectorParams1D=off
  q_des : Constant  Value=[0 1.2 0]
  v_des : Constant  Value=[0 0 0]
  w_des : Constant  Value=[0;0;0]  VectorParams1D=off
  refs : Outport
  wires:
  Bus Selector1/3 -> Bus Creator1/3  "<vz>"
  dw_des/1 -> Bus Creator2/4  "dw_des"
  Bus Selector1/2 -> Bus Creator1/2  "<vy>"
  q_des/1 -> Bus Creator2/1  "p_des"
  Bus Selector7/2 -> Bus Creator2/8  "<Q>"
  Bus Selector/3 -> Bus Creator/3  "<pz>"
  body states/1 -> Bus Selector7/1, Bus Selector1/1, Bus Selector/1
  Bus Selector1/1 -> Bus Creator1/1  "<vx>"
  v_des/1 -> Bus Creator2/2  "v_des"
  Bus Selector/1 -> Bus Creator/1  "<px>"
  Bus Creator/1 -> Bus Creator2/5  "p_cur"
  w_des/1 -> Bus Creator2/3  "w_des"
  Bus Selector/2 -> Bus Creator/2  "<py>"
  Bus Selector7/1 -> Bus Creator2/7  "<w>"
  Bus Creator1/1 -> Bus Creator2/6  "v_cur"
  Bus Creator2/1 -> refs/1

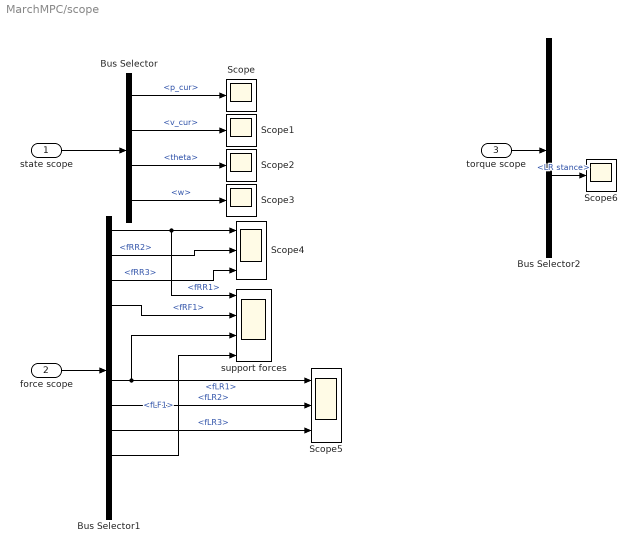
== system MarchMPC/scope ==
  state scope : Inport
  force scope : Inport  Port=2
  torque scope : Inport  Port=3
  Bus Selector : BusSelector  OutputSignals=p_cur,v_cur,theta,w
  Bus Selector1 : BusSelector  OutputSignals=fRR1,fRR2,fRR3,fRF1,fRF2,fRF3,fLR1,fLR2,fLR3,fLF1,fLF2,fLF3
  Bus Selector2 : BusSelector  OutputSignals=RR stance,RF stance,LR stance,LF stance
  Scope{,1..3,6} (5 alike) : Scope
  Scope4 : Scope  NumInputPorts=3
  Scope5 : Scope  NumInputPorts=3
  support forces : Scope  NumInputPorts=4
  wires:
  state scope/1 -> Bus Selector/1
  Bus Selector/1 -> Scope/1  "<p_cur>"
  Bus Selector/2 -> Scope1/1  "<v_cur>"
  Bus Selector/3 -> Scope2/1  "<theta>"
  Bus Selector/4 -> Scope3/1  "<w>"
  force scope/1 -> Bus Selector1/1
  Bus Selector1/1 -> support forces/1, Scope4/1  "<fRR1>"
  Bus Selector1/2 -> Scope4/2  "<fRR2>"
  Bus Selector1/3 -> Scope4/3  "<fRR3>"
  Bus Selector1/9 -> Scope5/3  "<fLR3>"
  Bus Selector1/8 -> Scope5/2  "<fLR2>"
  Bus Selector1/7 -> Scope5/1, support forces/3  "<fLR1>"
  torque scope/1 -> Bus Selector2/1
  Bus Selector2/3 -> Scope6/1  "<LR stance>"
  Bus Selector1/4 -> support forces/2  "<fRF1>"
  Bus Selector1/10 -> support forces/4  "<fLF1>"
